simulink model "Buoi_4"  (R2020b)
settings: Solver=VariableStepAuto  StartTime=0.0  StopTime=10.0  RelTol=1e-3
settings Model: Creator=long  LastModifiedBy=long

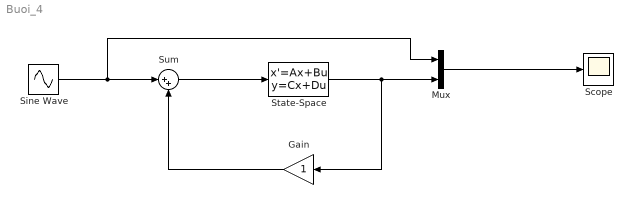
== system Buoi_4 ==
  Gain : Gain
  Mux : Mux  Inputs=2
  Scope : Scope
  Sine Wave : Sin  SampleTime=0
  State-Space : StateSpace  InitialCondition=0
  Sum : Sum  Inputs=|++
  wires:
  Mux/1 -> Scope/1
  State-Space/1 -> Gain/1, Mux/2
  Sum/1 -> State-Space/1
  Gain/1 -> Sum/2
  Sine Wave/1 -> Mux/1, Sum/1
